simulink model "SCo2"  (Simulink 8.5)
settings: Solver=ode23tb  SolverMode=SingleTasking  StartTime=0.0  StopTime=0.1  MaxStep=2e-4  RelTol=1e-3  AbsTol=1e-6
libraries: powerlib x100, powerlib_extras x21
(part 2 of 2)

== system SCo2/Original Three-phase system with a SLG Fault/Measuring Block/Three-Phase  Current Measurements/Current  Measurement2 ==
  Current Measurement1 : powerlib/Measurements/Current Measurement  PhasorSimulation=off  OutputType=Magnitude  PSBequivalent=0
  Fourier1 : powerlib_extras/Measurements/Fourier  f1=60  n=1
  Mux1 : Mux  Inputs=2
  + : PMIOPort  Port=1  Side=Left
  - : PMIOPort  Port=2  Side=Right
  Ip : Outport  InitialOutput=0
  I(t) : Outport  Port=2  InitialOutput=0
  wires:
  Fourier1/2 -> Mux1/2
  Fourier1/1 -> Mux1/1
  Mux1/1 -> Ip/1
  Current Measurement1/1 -> I(t)/1, Fourier1/1
  connections:
  +/RConn1 -- Current Measurement1/LConn1
  Current Measurement1/RConn1 -- -/RConn1
